simulink model "asbSkyHogg"  (R2023b)
settings: Solver=ode45  StartTime=0.0  StopTime=75  RelTol=1e-3  EnableMultiTasking=on
PreLoadFcn:
  | load asbSkyHoggData.mat
model workspace (MAT data in the model file):
  LatLong0 = [45 120]
  Sref = 20.9775
  Tc = 0.0166666666667
  Thrust = 2512.574
  Ts = 0
  V0 = 93.1047999839
  alpha0 = 0.0170924
  alt0 = 2000
  beta0 = 0
  bref = 12.5425
  cbar = 1.7526
  cg_0 = [2.158 0 0]
  g_0 = [0 0 9.81]
  heading0 = 0
  inertia = [5787.969  0  117.64; 0  6928.93  0; -117.64  0  11578.329]
  mass = 1299.21378662
  maxdef_aileron = 30
  maxdef_elevator = 20
  maxdef_rudder = 60
  mindef_aileron = -30
  mindef_elevator = -20
  mindef_rudder = -60
  mpoperpoint = opcond.OperatingPoint
  mpoperpoint.Version = 2
  mpoperpoint.Model_ = 'skyhogg3dof2V2'
  mpoperpoint.Time_ = 90
  mpoperpoint.States_(1) = opcond.StatePoint
  mpoperpoint.States_(1).Nx_ = 1
  mpoperpoint.States_(1).Block_ = 'skyhogg3dof2V2/Environment/Wind Models/Discrete Wind Gust Model/Distance into
    | gust (x)/Distance into
    | Gust (x)
    | (Limited to gust length d)'
  mpoperpoint.States_(2) = opcond.StatePoint
  mpoperpoint.States_(2).Nx_ = 1
  mpoperpoint.States_(2).Block_ = 'skyhogg3dof2V2/Environment/Wind Models/Discrete Wind Gust Model/Distance into
    | gust (y)/Distance into
    | Gust (x)
    | (Limited to gust length d)
    | '
  mpoperpoint.States_(3) = opcond.StatePoint
  mpoperpoint.States_(3).Nx_ = 1
  mpoperpoint.States_(3).Block_ = 'skyhogg3dof2V2/Environment/Wind Models/Discrete Wind Gust Model/Distance into
    | gust (z)/Distance into
    | Gust (x)
    | (Limited to gust length d)
    | '
  mpoperpoint.States_(4) = opcond.StatePoint
  mpoperpoint.States_(4).Nx_ = 2
  mpoperpoint.States_(4).Block_ = 'skyhogg3dof2V2/Environment/Wind Models/Dryden Wind Turbulence Model 
    | (Continuous (+q +r))/Filters on angular rates/Hpgw/pgw_p'
  mpoperpoint.States_(4).x_ = [0; 0]
  mpoperpoint.States_(5) = opcond.StatePoint
  mpoperpoint.States_(5).Nx_ = 2
  mpoperpoint.States_(5).Block_ = 'skyhogg3dof2V2/Environment/Wind Models/Dryden Wind Turbulence Model 
    | (Continuous (+q +r))/Filters on angular rates/Hqgw/qgw_p'
  mpoperpoint.States_(5).x_ = [0; 0]
  mpoperpoint.States_(6) = opcond.StatePoint
  mpoperpoint.States_(6).Nx_ = 2
  mpoperpoint.States_(6).Block_ = 'skyhogg3dof2V2/Environment/Wind Models/Dryden Wind Turbulence Model 
    | (Continuous (+q +r))/Filters on angular rates/Hrgw/rgw_p'
  mpoperpoint.States_(6).x_ = [0; 0]
  mpoperpoint.States_(7) = opcond.StatePoint
  mpoperpoint.States_(7).Nx_ = 2
  mpoperpoint.States_(7).Block_ = 'skyhogg3dof2V2/Environment/Wind Models/Dryden Wind Turbulence Model 
    | (Continuous (+q +r))/Filters on velocities/Hugw(s)/ug_p'
  mpoperpoint.States_(7).x_ = [0; 0]
  mpoperpoint.States_(8) = opcond.StatePoint
  mpoperpoint.States_(8).Nx_ = 2
  mpoperpoint.States_(8).Block_ = 'skyhogg3dof2V2/Environment/Wind Models/Dryden Wind Turbulence Model 
    | (Continuous (+q +r))/Filters on velocities/Hvgw(s)/vg_p1'
  mpoperpoint.States_(8).x_ = [0; 0]
  mpoperpoint.States_(9) = opcond.StatePoint
  mpoperpoint.States_(9).Nx_ = 2
  mpoperpoint.States_(9).Block_ = 'skyhogg3dof2V2/Environment/Wind Models/Dryden Wind Turbulence Model 
    | (Continuous (+q +r))/Filters on velocities/Hvgw(s)/vgw_p2'
  mpoperpoint.States_(9).x_ = [0; 0]
  mpoperpoint.States_(10) = opcond.StatePoint
  mpoperpoint.States_(10).Nx_ = 2
  mpoperpoint.States_(10).Block_ = 'skyhogg3dof2V2/Environment/Wind Models/Dryden Wind Turbulence Model 
    | (Continuous (+q +r))/Filters on velocities/Hwgw(s)/wg_p1'
  mpoperpoint.States_(10).x_ = [0; 0]
  mpoperpoint.States_(11) = opcond.StatePoint
  mpoperpoint.States_(11).Nx_ = 2
  mpoperpoint.States_(11).Block_ = 'skyhogg3dof2V2/Environment/Wind Models/Dryden Wind Turbulence Model 
    | (Continuous (+q +r))/Filters on velocities/Hwgw(s)/wg_p2'
  mpoperpoint.States_(11).x_ = [0; 0]
  mpoperpoint.States_(12) = opcond.StatePoint
  mpoperpoint.States_(12).Nx_ = 1
  mpoperpoint.States_(12).Block_ = 'skyhogg3dof2V2/Pilot/Zero-Pole'
  mpoperpoint.States_(12).x_ = 100
  mpoperpoint.States_(13) = opcond.StatePoint
  mpoperpoint.States_(13).Nx_ = 3
  mpoperpoint.States_(13).Block_ = 'skyhogg3dof2V2/Vehicle System Model/Avionics/Autopilot/Alt Controller'
  mpoperpoint.States_(13).x_ = [3773.13420468; 1565572.17222; 1483525.59759]
  mpoperpoint.States_(13).Ts_ = [0.0166666666667 0]
  mpoperpoint.States_(13).SampleType_ = 'DSTATE'
  mpoperpoint.States_(14) = opcond.StatePoint
  mpoperpoint.States_(14).Nx_ = 2
  mpoperpoint.States_(14).Block_ = 'skyhogg3dof2V2/Vehicle System Model/Avionics/Autopilot/Theata Controller'
  mpoperpoint.States_(14).x_ = [2.75911094331; 0.799199587737]
  mpoperpoint.States_(14).Ts_ = [0.0166666666667 0]
  mpoperpoint.States_(14).SampleType_ = 'DSTATE'
  mpoperpoint.States_(15) = opcond.StatePoint
  mpoperpoint.States_(15).Nx_ = 2
  mpoperpoint.States_(15).Block_ = 'skyhogg3dof2V2/Vehicle System Model/Avionics/Autopilot/Zero-Pole'
  mpoperpoint.States_(15).x_ = [-4.06142023407e-07; 20.0015832662]
  mpoperpoint.States_(16) = opcond.StatePoint
  mpoperpoint.States_(16).Nx_ = 2
  mpoperpoint.States_(16).Block_ = 'skyhogg3dof2V2/Vehicle System Model/Avionics/Three-axis IMU/Three-axis Accelerometer/Dynamics/Second-order Dynamics/Transfer Fcn X/Discrete
    | Transfer Fcn'
  mpoperpoint.States_(16).x_ = [0; 0]
  mpoperpoint.States_(16).Ts_ = [0.0166666666667 0]
  mpoperpoint.States_(16).SampleType_ = 'DSTATE'
  mpoperpoint.States_(17) = opcond.StatePoint
  mpoperpoint.States_(17).Nx_ = 2
  mpoperpoint.States_(17).Block_ = 'skyhogg3dof2V2/Vehicle System Model/Avionics/Three-axis IMU/Three-axis Accelerometer/Dynamics/Second-order Dynamics/Transfer Fcn Y/Discrete
    | Transfer Fcn'
  mpoperpoint.States_(17).x_ = [0; 0]
  mpoperpoint.States_(17).Ts_ = [0.0166666666667 0]
  mpoperpoint.States_(17).SampleType_ = 'DSTATE'
  mpoperpoint.States_(18) = opcond.StatePoint
  mpoperpoint.States_(18).Nx_ = 2
  mpoperpoint.States_(18).Block_ = 'skyhogg3dof2V2/Vehicle System Model/Avionics/Three-axis IMU/Three-axis Accelerometer/Dynamics/Second-order Dynamics/Transfer Fcn Z/Discrete
    | Transfer Fcn'
  mpoperpoint.States_(18).x_ = [0; 0]
  mpoperpoint.States_(18).Ts_ = [0.0166666666667 0]
  mpoperpoint.States_(18).SampleType_ = 'DSTATE'
  mpoperpoint.States_(19) = opcond.StatePoint
  mpoperpoint.States_(19).Nx_ = 2
  mpoperpoint.States_(19).Block_ = 'skyhogg3dof2V2/Vehicle System Model/Avionics/Three-axis IMU/Three-axis Gyroscope/Dynamics/Second-order Dynamics/Transfer Fcn X/Discrete
    | Transfer Fcn'
  mpoperpoint.States_(19).x_ = [0; 0]
  mpoperpoint.States_(19).Ts_ = [0.0166666666667 0]
  mpoperpoint.States_(19).SampleType_ = 'DSTATE'
  mpoperpoint.States_(20) = opcond.StatePoint
  mpoperpoint.States_(20).Nx_ = 2
  mpoperpoint.States_(20).Block_ = 'skyhogg3dof2V2/Vehicle System Model/Avionics/Three-axis IMU/Three-axis Gyroscope/Dynamics/Second-order Dynamics/Transfer Fcn Y/Discrete
    | Transfer Fcn'
  mpoperpoint.States_(20).x_ = [0; 0]
  mpoperpoint.States_(20).Ts_ = [0.0166666666667 0]
  mpoperpoint.States_(20).SampleType_ = 'DSTATE'
  mpoperpoint.States_(21) = opcond.StatePoint
  mpoperpoint.States_(21).Nx_ = 2
  mpoperpoint.States_(21).Block_ = 'skyhogg3dof2V2/Vehicle System Model/Avionics/Three-axis IMU/Three-axis Gyroscope/Dynamics/Second-order Dynamics/Transfer Fcn Z/Discrete
    | Transfer Fcn'
  mpoperpoint.States_(21).x_ = [0; 0]
  mpoperpoint.States_(21).Ts_ = [0.0166666666667 0]
  mpoperpoint.States_(21).SampleType_ = 'DSTATE'
  mpoperpoint.States_(22) = opcond.StatePoint
  mpoperpoint.States_(22).Nx_ = 2
  mpoperpoint.States_(22).Block_ = 'skyhogg3dof2V2/Vehicle System Model/Vehicle/3DoF to 6DoF/3DoF (Body Axes)/Position'
  mpoperpoint.States_(22).x_ = [8095.191026; -2000.15815038]
  mpoperpoint.States_(23) = opcond.StatePoint
  mpoperpoint.States_(23).Nx_ = 1
  mpoperpoint.States_(23).Block_ = 'skyhogg3dof2V2/Vehicle System Model/Vehicle/3DoF to 6DoF/3DoF (Body Axes)/Theta'
  mpoperpoint.States_(23).x_ = 0.017215052061
  mpoperpoint.States_(24) = opcond.StatePoint
  mpoperpoint.States_(24).Nx_ = 2
  mpoperpoint.States_(24).Block_ = 'skyhogg3dof2V2/Vehicle System Model/Vehicle/3DoF to 6DoF/3DoF (Body Axes)/U,w'
  mpoperpoint.States_(24).x_ = [92.5982047244; 1.60074325578]
  mpoperpoint.States_(25) = opcond.StatePoint
  mpoperpoint.States_(25).Nx_ = 1
  mpoperpoint.States_(25).Block_ = 'skyhogg3dof2V2/Vehicle System Model/Vehicle/3DoF to 6DoF/3DoF (Body Axes)/q'
  mpoperpoint.States_(25).x_ = -4.72902107138e-06
  mpoperpoint.States_(26) = opcond.StatePoint
  mpoperpoint.States_(26).Nx_ = 1
  mpoperpoint.States_(26).Block_ = 'skyhogg3dof2V2/Vehicle System Model/Vehicle/AirframeActuators/2nd Order Non-linear Actuator/Limited
    | Deflection'
  mpoperpoint.States_(27) = opcond.StatePoint
  mpoperpoint.States_(27).Nx_ = 1
  mpoperpoint.States_(27).Block_ = 'skyhogg3dof2V2/Vehicle System Model/Vehicle/AirframeActuators/2nd Order Non-linear Actuator/Servo rate'
  mpoperpoint.States_(28) = opcond.StatePoint
  mpoperpoint.States_(28).Nx_ = 1
  mpoperpoint.States_(28).Block_ = 'skyhogg3dof2V2/Vehicle System Model/Vehicle/AirframeActuators/2nd Order Non-linear Actuator1/Limited
    | Deflection'
  mpoperpoint.States_(28).x_ = -1.01356346376
  mpoperpoint.States_(29) = opcond.StatePoint
  mpoperpoint.States_(29).Nx_ = 1
  mpoperpoint.States_(29).Block_ = 'skyhogg3dof2V2/Vehicle System Model/Vehicle/AirframeActuators/2nd Order Non-linear Actuator1/Servo rate'
  mpoperpoint.States_(29).x_ = 0.00390789331449
  mpoperpoint.States_(30) = opcond.StatePoint
  mpoperpoint.States_(30).Nx_ = 1
  mpoperpoint.States_(30).Block_ = 'skyhogg3dof2V2/Vehicle System Model/Vehicle/AirframeActuators/2nd Order Non-linear Actuator2/Limited
    | Deflection'
  mpoperpoint.States_(31) = opcond.StatePoint
  mpoperpoint.States_(31).Nx_ = 1
  mpoperpoint.States_(31).Block_ = 'skyhogg3dof2V2/Vehicle System Model/Vehicle/AirframeActuators/2nd Order Non-linear Actuator2/Servo rate'
  theta0 = 0.017092
  wn_act = 44
  wy0 = 0
  z_act = 0.7
undefined symbols (not defined in the file): F, Light, MIL, pa28, thottleValue
libraries: aerolibwind2 x3, aerolibfltsims x2, aerolibatmos2 x1, simulink x1, simulink_extras x1
Description:
  | Lightweight Airplane Design
  | 
  | This is the three degree-of-freedom model of a lightweight four-seater
  | low wing monoplane with a longitudinal autopilot.
settings Model: DataDictionary=asdSkyHogg_Data.sldd  Creator=The MathWorks, Inc.  LastModifiedBy=Gamax
settings SolverCC: AlgebraicLoopSolver=TrustRegion  MaxZcPerStep=1
settings DataIOCC: ExternalInput=getinputstruct(op_skyhogg3dof2V5)  InitialState=getstatestruct(op_skyhogg3dof2V5)  LimitDataPoints=on  SaveFormat=StructureWithTime  ReturnWorkspaceOutputs=off
settings OptimizationCC: BlockReduction=off  BufferReuse=off  ExpressionDepthLimit=2147483647  InitFltsAndDblsToZero=on  LifeSpan=inf
settings DebuggingCC: WriteAfterWriteMsg=DisableAll  AlgebraicLoopMsg=none  SaveWithParameterizedLinksMsg=none  SignalResolutionControl=TryResolveAllWithWarning  FcnCallInpInsideContextMsg=warning  UniqueDataStoreMsg=error  AllowSymbolicDim=off  StateNameClashWarn=warning  SubsystemReferenceDiagnosticForUnitTest=warning  StrictBusMsg=ErrorOnBusTreatedAsVector  SFUnexpectedBacktrackingDiag=warning  SFNoUnconditionalDefaultTransitionDiag=warning  SFExecutionAtInitializationDiag=none  ArithmeticOperatorsInVariantConditions=warning
settings HardwareCC: ProdBitPerPointer=32  ProdBitPerSizeT=32  ProdBitPerPtrDiffT=32  ProdLargestAtomicFloat=None  ProdIntDivRoundTo=Undefined  ProdEndianess=Unspecified  ProdWordSize=32  ProdHWDeviceType=32-bit Generic
settings ModelReferenceCC: EnableRefExpFcnMdlSchedulingChecks=on  PropagateSignalLabelsOutOfModel=off
settings SFSimCC: SimUseLocalCustomCode=off  CustomCodeUndefinedFunction=UseInterfaceOnly
settings RTWCC: RTWUseLocalCustomCode=off  DLArmComputeVersion=19.05
settings CodeAppCC: StateflowObjectComments=on
settings GRTTargetCC: TargetFcnLib=ansi_tfl_tmw.mat  TargetLangStandard=C89/C90 (ANSI)  CombineOutputUpdateFcns=off  GRTInterface=on
settings ConfigComp: CovMetricSettings=dw  CovSaveCumulativeToWorkspaceVar=on  CovSaveSingleToWorkspaceVar=on  CovExternalEMLEnable=off  CovSFcnEnable=off

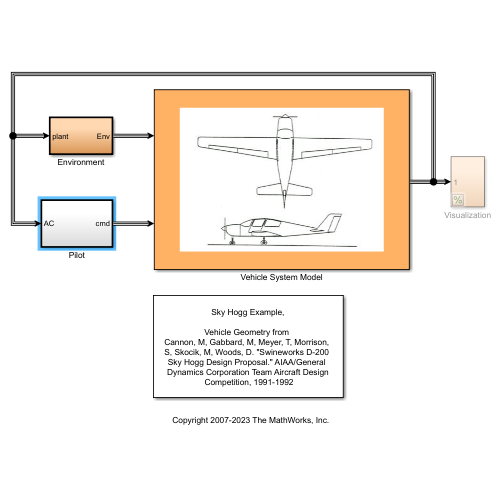
[thumbnail: Simulink's stored preview of the top-level diagram]
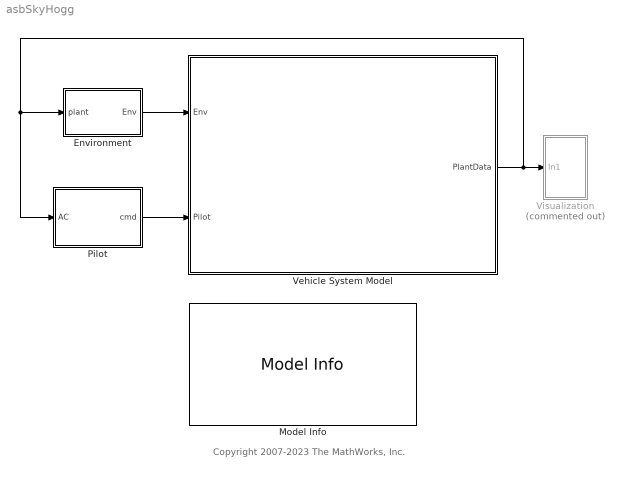
== system asbSkyHogg ==
  note: Copyright 2007-2023 The MathWorks, Inc.
  Environment : Subsystem  TreatAsAtomicUnit=on
  Model Info : simulink/Model-Wide Utilities/Model Info  Frame=on  DisplayStringWithTags=|  HorizontalTextAlignment=Center  LeftAlignmentValue=0.5
      | Sky Hogg Example,
      | 
      | Vehicle Geometry from 
      | Cannon, M, Gabbard, M, Meyer, T, Morrison, 
      | S, Skocik, M, Woods, D. "Swineworks D-200 
      | Sky Hogg Design Proposal." AIAA/General 
      | Dynamics Corporation Team Aircraft Design
      |  Competition, 1991-1992
  Pilot : Subsystem  TreatAsAtomicUnit=on
  Vehicle System Model : Subsystem
      mask Display: image('asbSkyHogg.jpg',[.1 .1 .8 .8],'on')
  Visualization : Subsystem  Commented=on
  wires:
  Environment/1(Env) -> Vehicle System Model/1(Env)
  Vehicle System Model/1(PlantData) -> Environment/1(plant), Pilot/1(AC), Visualization/1(In1)
  Pilot/1(cmd) -> Vehicle System Model/2(Pilot)

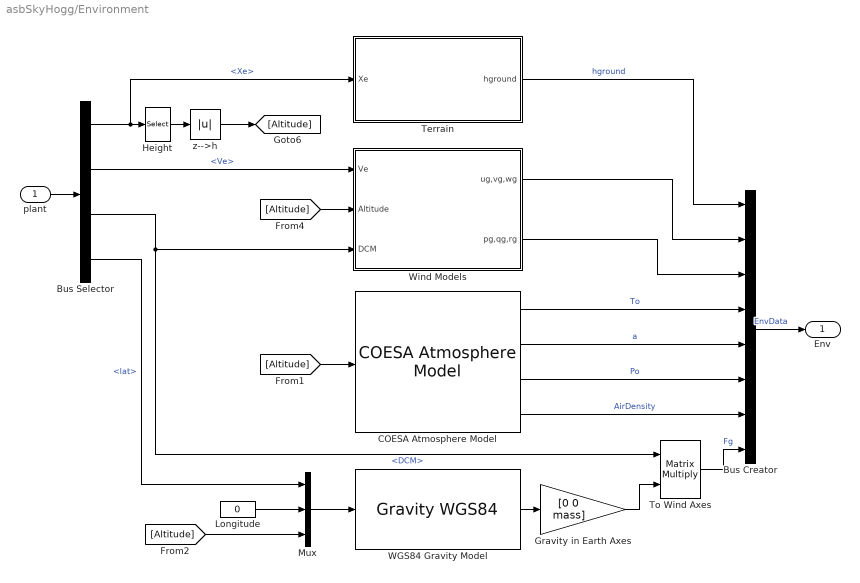
== system asbSkyHogg/Environment ==
  plant : Inport
  Bus Creator : BusCreator  Inputs='hground','WindVelocity','WindAngularRates','To','a','Po','AirDensity','Fg'
  Bus Selector : BusSelector  OutputSignals=Xe,Ve,DCM,lat
  COESA Atmosphere Model : aerolibatmos2/COESA Atmosphere Model  units=Metric (MKS)  spec=1976 COESA-extended U.S. Standard Atmosphere  model=Profile  profile_var=High temperature  profile_percent=1%  profile_alt=5 km (16404 ft)  envelope_var=High temperature  envelope_percent=1%  action=Warning
  Gravity in Earth Axes : Gain  Gain=[0 0 mass]  SaturateOnIntegerOverflow=on  OutDataTypeStr=Inherit: Same as input  ParamDataTypeStr=Inherit: Same as input
  Height : Selector  IndexMode=Zero-based  InputPortWidth=3  IndexOptions=Index vector (dialog)  Indices=2  OutputSizes=1
  Longitude : Constant  Value=0
  Mux : Mux  Inputs=3
  Terrain : Subsystem
  To Wind Axes : Product  Multiplication=Matrix(*)  InputSameDT=on  SaturateOnIntegerOverflow=on  OutDataTypeStr=Inherit: Same as first input
  "WGS84 Gravity Model  " : GravityWGS84
  Wind Models : Subsystem
  z-->h : Abs
  Env : Outport  InitialOutput=0  VectorParamsAs1DForOutWhenUnconnected=off
  wires:
  Bus Selector/3 -> To Wind Axes/1, Wind Models/3(DCM)  "<DCM>"
  Bus Selector/2 -> Wind Models/1(Ve)  "<Ve>"
  Bus Selector/1 -> Height/1, Terrain/1(Xe)  "<Xe>"
  [Altitude] -> COESA Atmosphere Model/1
  [Altitude] -> Mux/3
  [Altitude] -> Wind Models/2(Altitude)
  z-->h/1 -> [Altitude]
  plant/1 -> Bus Selector/1
  Bus Creator/1 -> Env/1  "EnvData"
  To Wind Axes/1 -> Bus Creator/8  "Fg"
  Gravity in Earth Axes/1 -> To Wind Axes/2
  "WGS84 Gravity Model  "/1 -> Gravity in Earth Axes/1
  Bus Selector/4 -> Mux/1  "<lat>"
  Height/1 -> z-->h/1
  COESA Atmosphere Model/1 -> Bus Creator/4  "To"
  COESA Atmosphere Model/3 -> Bus Creator/6  "Po"
  COESA Atmosphere Model/2 -> Bus Creator/5  "a"
  COESA Atmosphere Model/4 -> Bus Creator/7  "AirDensity"
  Wind Models/2(pg,qg,rg) -> Bus Creator/3
  Wind Models/1(ug,vg,wg) -> Bus Creator/2
  Terrain/1(hground) -> Bus Creator/1  "hground"
  Mux/1 -> "WGS84 Gravity Model  "/1
  Longitude/1 -> Mux/2

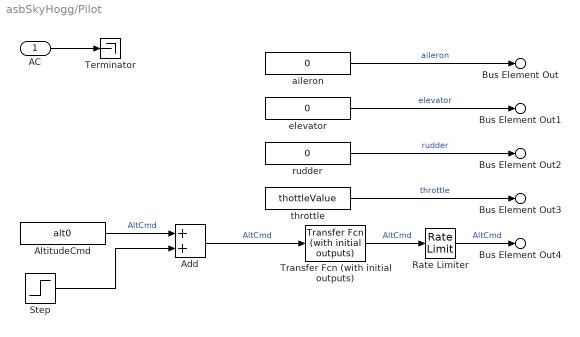
== system asbSkyHogg/Pilot ==
  AC : Inport
  Add : Sum
  AltitudeCmd : Constant  Value=alt0  OutDataTypeStr=double
  Rate Limiter : RateLimiter  RisingSlewLimit=500/3/60  SampleTimeMode=inherited  InitialCondition=2000
  Step : Step  Time=5  After=50  SampleTime=0
  Terminator : Terminator
  Transfer Fcn (with initial outputs) : simulink_extras/Additional Linear/Transfer Fcn (with initial outputs)  N=.25  D=[1,.25]  Y0=2000  U0=2000
  aileron : Constant  Value=0  OutDataTypeStr=single
  elevator : Constant  Value=0  OutDataTypeStr=single
  rudder : Constant  Value=0  OutDataTypeStr=single
  throttle : Constant  Value=thottleValue  OutDataTypeStr=double
  Bus Element Out : Outport  PortName=cmd  Element=aileron
  Bus Element Out1 : Outport  PortName=cmd  Element=elevator
  Bus Element Out3 : Outport  PortName=cmd  Element=throttle
  Bus Element Out4 : Outport  PortName=cmd  Element=AltCmd
  Bus Element Out2 : Outport  PortName=cmd  Element=rudder
  wires:
  aileron/1 -> Bus Element Out/1  "aileron"
  AC/1 -> Terminator/1
  AltitudeCmd/1 -> Add/1  "AltCmd"
  Step/1 -> Add/2
  Add/1 -> Transfer Fcn (with initial outputs)/1  "AltCmd"
  Rate Limiter/1 -> Bus Element Out4/1  "AltCmd"
  Transfer Fcn (with initial outputs)/1 -> Rate Limiter/1  "AltCmd"
  elevator/1 -> Bus Element Out1/1  "elevator"
  rudder/1 -> Bus Element Out2/1  "rudder"
  throttle/1 -> Bus Element Out3/1  "throttle"

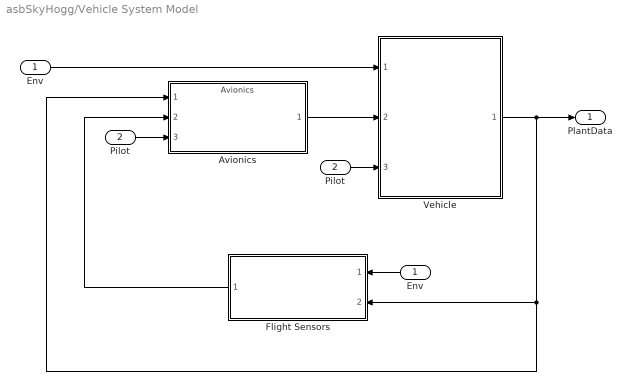
== system asbSkyHogg/Vehicle System Model ==
  Env : Inport
  Pilot : Inport  Port=2  OutDataTypeStr=Bus: PilotCmdBus
  Avionics : ModelReference  ModelNameDialog=Avionics  SimulationMode=Normal  ModelReferenceVersion=10.47
  "Env " : InportShadow
  Flight Sensors : Subsystem  ReferencedSubsystem=Flight_Sensors
  "Pilot " : InportShadow  Port=2  OutDataTypeStr=Bus: PilotCmdBus
  Vehicle : Subsystem  ReferencedSubsystem=Vehicle
  PlantData : Outport  VectorParamsAs1DForOutWhenUnconnected=off
  wires:
  Env/1 -> Vehicle/1
  Vehicle/1 -> PlantData/1, Flight Sensors/2, Avionics/1
  Flight Sensors/1 -> Avionics/2
  Avionics/1 -> Vehicle/2
  Pilot/1 -> Vehicle/3
  "Env "/1 -> Flight Sensors/1
  "Pilot "/1 -> Avionics/3

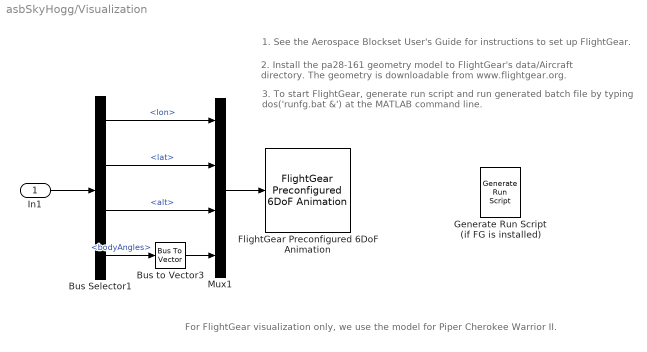
== system asbSkyHogg/Visualization ==
  note: For FlightGear visualization only, we use the model for Piper Cherokee Warrior II.
  note: 3. To start FlightGear, generate run script and run generated batch file by typing
      |      dos('runfg.bat &') at the MATLAB command line.
  note: 1. See the Aerospace Blockset User's Guide for instructions to set up FlightGear.
  note: 2. Install the pa28-161 geometry model to FlightGear's data/Aircraft
      |     directory. The geometry is downloadable from www.flightgear.org.
  In1 : Inport
  Bus Selector1 : BusSelector  OutputSignals=lon,lat,alt,bodyAngles
  Bus to Vector3 : BusToVector
  FlightGear Preconfigured 6DoF Animation : aerolibfltsims/FlightGear Preconfigured 6DoF Animation  xFlightGearVersion=v2019.1  DestinationIpAddress=127.0.0.1  DestinationPort=5502  SampleTime=1/30  packetVersion=24
  Generate Run Script (if FG is installed) : aerolibfltsims/Generate Run Script  Architecture=Default  dataFlow=Send  GeometryModelName=pa28-161  AirportId=KSFO  RunwayId=10L  InitialAltitude=7224  InitialHeading=113  OffsetDistance=4.72  OffsetAzimuth=0  InstallScenery=on  DisableShaders=on  OriginAddress=127.0.0.1  DestinationPort=5502  OriginPort=5505  LocalAddress=127.0.0.1  OutputFileName=runfg.bat  FlightGearBaseDirectory=C:\Program Files\FlightGear
  Mux1 : Mux
  wires:
  In1/1 -> Bus Selector1/1
  Bus Selector1/1 -> Mux1/1  "<lon>"
  Bus Selector1/2 -> Mux1/2  "<lat>"
  Bus Selector1/3 -> Mux1/3  "<alt>"
  Bus Selector1/4 -> Bus to Vector3/1  "<bodyAngles>"
  Mux1/1 -> FlightGear Preconfigured 6DoF Animation/1
  Bus to Vector3/1 -> Mux1/4

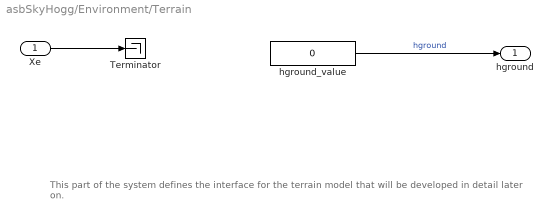
== system asbSkyHogg/Environment/Terrain ==
  note: This part of the system defines the interface for the terrain model that will be developed in detail later on.
  Xe : Inport
  Terminator : Terminator
  hground_value : Constant  Value=0  OutDataTypeStr=single
  hground : Outport  Unit=m  VectorParamsAs1DForOutWhenUnconnected=off
  wires:
  hground_value/1 -> hground/1  "hground"
  Xe/1 -> Terminator/1

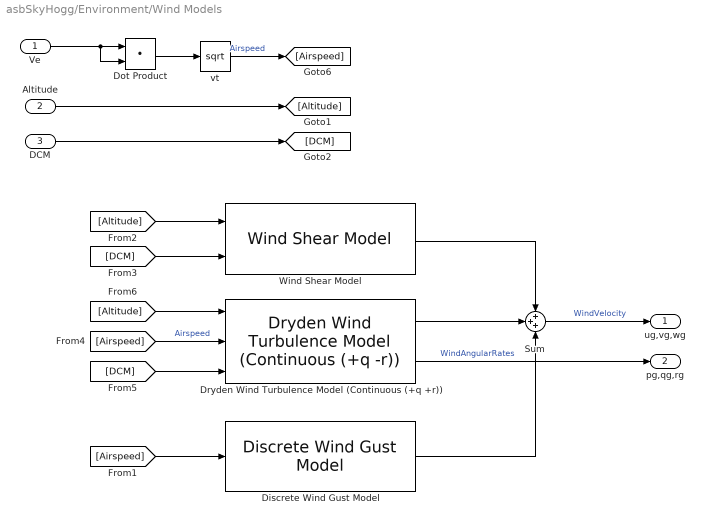
== system asbSkyHogg/Environment/Wind Models ==
  Ve : Inport
  Altitude : Inport  Port=2
  DCM : Inport  Port=3
  Discrete Wind Gust Model : aerolibwind2/Discrete Wind Gust Model  units=Metric (MKS)  Gx=off  Gy=off  Gz=off  t_0=20  d_m=[120 120 80]  v_m=[3.5 3.0 3.0]
  Dot Product : DotProduct  InputSameDT=off  OutDataTypeStr=Inherit: Inherit via internal rule
  Dryden Wind Turbulence Model (Continuous (+q +r)) : aerolibwind2/Dryden Wind Turbulence Model  (Continuous (+q -r))  units=Metric (MKS)  spec=MIL-F-8785C  model=Continuous Dryden (+q +r)  W20=5  Wdeg=0  TurbProb=10^-2 - Light  L_high=533.4  Wingspan=4  ts=0.1  Seed=[23341 23342 23343 23344]  T_on=off
  Sum : Sum  Inputs=+++  InputSameDT=on  SaturateOnIntegerOverflow=on  OutDataTypeStr=Inherit: Same as first input
  Wind Shear Model : aerolibwind2/Wind Shear Model  units=Metric (MKS)  phase=Category C - Terminal Flight Phase  W_20=1  Wdeg=0
  vt : Sqrt
  ug,vg,wg : Outport  Unit=m/s  VectorParamsAs1DForOutWhenUnconnected=off
  pg,qg,rg : Outport  Port=2  Unit=rad/second  VectorParamsAs1DForOutWhenUnconnected=off
  wires:
  [Altitude] -> Dryden Wind Turbulence Model (Continuous (+q +r))/1
  [DCM] -> Dryden Wind Turbulence Model (Continuous (+q +r))/3
  [DCM] -> Wind Shear Model/2
  DCM/1 -> [DCM]
  [Altitude] -> Wind Shear Model/1
  Altitude/1 -> [Altitude]
  [Airspeed] -> Discrete Wind Gust Model/1
  vt/1 -> [Airspeed]  "Airspeed"
  Dot Product/1 -> vt/1
  Dryden Wind Turbulence Model (Continuous (+q +r))/2 -> pg,qg,rg/1  "WindAngularRates"
  [Airspeed] -> Dryden Wind Turbulence Model (Continuous (+q +r))/2  "Airspeed"
  Sum/1 -> ug,vg,wg/1  "WindVelocity"
  Discrete Wind Gust Model/1 -> Sum/3
  Dryden Wind Turbulence Model (Continuous (+q +r))/1 -> Sum/2
  Wind Shear Model/1 -> Sum/1
  Ve/1 -> Dot Product/2, Dot Product/1
